simulink model "sldemo_bumpless"  (Simulink 7.6)
settings: Solver=ode45  StartTime=0.0  StopTime=600  MaxStep=0.1  RelTol=1e-5
undefined symbols (not defined in the file): sigbuilder_block
libraries: simulink x2
settings Model: Creator=The MathWorks Inc.

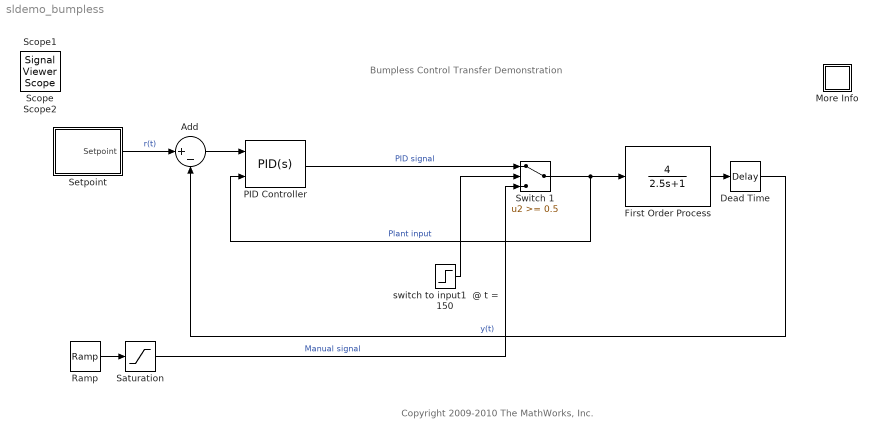
== system sldemo_bumpless ==
  note: Bumpless Control Transfer Demonstration
  note: Copyright 2009-2010 The MathWorks, Inc.
  Add : Sum  Inputs=|+-
  Dead Time : TransportDelay  BufferSize=2048
  First Order Process : TransferFcn  Numerator=4  Denominator=[2.5 1]
  More Info : Subsystem
      settings: OpenFcn=showdemo('sldemo_bumpless')
      mask Display: disp('?')
  PID Controller : simulink/Continuous/PID Controller  DialogController=pidpack.PIDConfig.pidDDGCreate  DialogControllerArgs=DataTag0  SystemSampleTime=-1  Controller=PID  TimeDomain=Continuous-time  SampleTime=1  IntegratorMethod=Forward Euler  FilterMethod=Forward Euler  Form=Parallel  P=0.32051437453006  I=0.13025295582387  D=0  N=100  InitialConditionSource=internal  InitialConditionForIntegrator=0  InitialConditionForFilter=0  ExternalReset=none  LimitOutput=off  UpperSaturationLimit=inf  LowerSaturationLimit=-inf  LinearizeAsGain=off  AntiWindupMode=none  Kb=1  TrackingMode=on  Kt=1  PParamMin=[]  PParamMax=[]  IParamMin=[]  IParamMax=[]  DParamMin=[]  DParamMax=[]  NParamMin=[]  NParamMax=[]  KbParamMin=[]  KbParamMax=[]  KtParamMin=[]  KtParamMax=[]  POutMin=[]  POutMax=[]  IOutMin=[]  IOutMax=[]  DOutMin=[]  DOutMax=[]  NOutMin=[]  NOutMax=[]  KbOutMin=[]  KbOutMax=[]  KtOutMin=[]  KtOutMax=[]  IntegratorOutMin=[]  IntegratorOutMax=[]  FilterOutMin=[]  FilterOutMax=[]  SumOutMin=[]  SumOutMax=[]  SumI1OutMin=[]  SumI1OutMax=[]  SumI2OutMin=[]  SumI2OutMax=[]  SumI3OutMin=[]  SumI3OutMax=[]  SumDOutMin=[]  SumDOutMax=[]  SaturationOutMin=[]  SaturationOutMax=[]  IntegratorContinuousStateAttributes=''  IntegratorStateMustResolveToSignalObject=off  IntegratorRTWStateStorageClass=Auto  FilterContinuousStateAttributes=''  FilterStateMustResolveToSignalObject=off  FilterRTWStateStorageClass=Auto
  Ramp : simulink/Sources/Ramp  SystemSampleTime=-1  slope=0.1  start=0  X0=0
  Saturation : Saturate  UpperLimit=10  LowerLimit=-10
  Setpoint : Subsystem  Tag=STV Subsys  LoadFcn=sigbuilder_block('load');  StartFcn=sigbuilder_block('start');  StopFcn=sigbuilder_block('stop');  ClipboardFcn=sigbuilder_block('clipboard');  mask(Sigbuilder block){}
      mask help: Create and generate interchangeable groups of signals whose waveforms are piecewise linear.
      mask init:
      | if ~strcmp(get_param(bdroot(gcbh),'SimulationStatus'),'stopped') tuvar = sigbuilder_block('maskInit'); end
      settings: CopyFcn=sigbuilder_block('copy');  DeleteFcn=sigbuilder_block('delete');  ModelCloseFcn=sigbuilder_block('modelClose');  PreSaveFcn=sigbuilder_block('preSave');  NameChangeFcn=sigbuilder_block('namechange');  OpenFcn=sigbuilder_block('open',[332.25 289.5 550.5 399.75 ]);  CloseFcn=sigbuilder_block('close');
      mask Display: plot(0,0,100,100,[10,10,40,40,10],[80,20,20,80,80],[40,10],[50,50], [40,27,10],[65,72,56],[40,25,25,10],[28,28,43,43]);
  Switch 1 : Switch  Threshold=0.5
  switch to input1  @ t = 150 : Step  Time=150  SampleTime=0
  Scope : SignalViewerScope  IOType=viewer  LegendLocations="322.3333      286.3333            72            36"  RefreshTime=0.035000
      settings: ShowLegends=on  TimeRange=600  YMin=0  YMax=50  MaxDataPoints=100000
  Scope1 : SignalViewerScope  IOType=viewer  LegendLocations="270.3333      282.3333           123            36"  RefreshTime=0.035000
      settings: ShowLegends=on  TimeRange=600  YMin=0  YMax=12  MaxDataPoints=100000
  Scope2 : SignalViewerScope  IOType=viewer  LegendLocations="286.3333           298           108      20.33333"  RefreshTime=0.035000
      settings: ShowLegends=on  TimeRange=600  YMin=0  YMax=12  SaveName=ScopeData2  MaxDataPoints=100000
  wires:
  Add/1 -> PID Controller/1
  Dead Time/1 -> Add/2  "y(t)"
  Switch 1/1 -> First Order Process/1, PID Controller/2  "Plant input"
  PID Controller/1 -> Switch 1/1  "PID signal"
  Saturation/1 -> Switch 1/3  "Manual signal"
  Setpoint/1(Setpoint) -> Add/1  "r(t)"
  First Order Process/1 -> Dead Time/1
  switch to input1  @ t = 150/1 -> Switch 1/2
  Ramp/1 -> Saturation/1

== system sldemo_bumpless/More Info ==

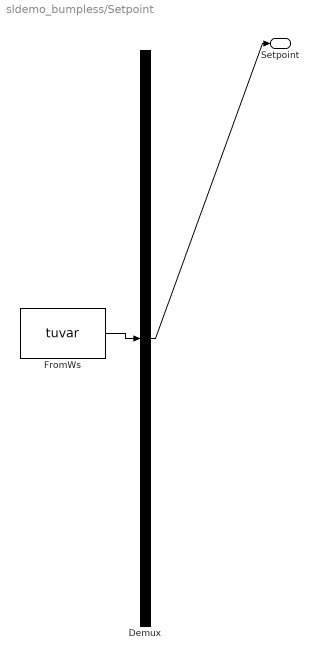
== system sldemo_bumpless/Setpoint ==
  Demux : Demux  Tag=STV Demux  Outputs=1
  FromWs : FromWorkspace  Tag=STV FromWs  VariableName=tuvar  SampleTime=0  SigBuilderData=DataTag1  VnvData=DataTag2
      SigBuilderData=|
      | common.afterFinalStr = 'Extrapolate'
      | common.sampleTime = 0
      | dataSet.timeRange = [0 800]
      | dataSet.name = 'Group 1'
      | sbobj.Groups.Name = 'Group 1'
      | sbobj.Groups.Signals.Name = 'Setpoint'
      | sbobj.Groups.Signals.XData = [0 320 480 800]
      | sbobj.Groups.Signals.YData = [40 40 20 20]
  Setpoint : Outport  Tag=STV Outport
  wires:
  FromWs/1 -> Demux/1
  Demux/1 -> Setpoint/1
